simulink model "prob1"  (R2020b)
settings: Solver=VariableStepAuto  StartTime=0.0  StopTime=inf  RelTol=1e-3
settings Model: Creator=HP  LastModifiedBy=Admin

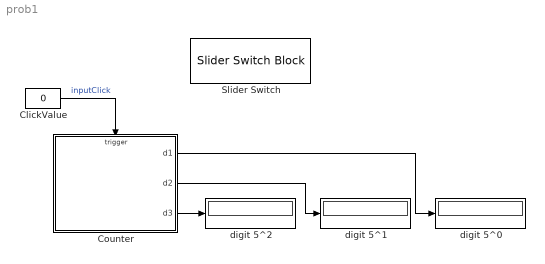
== system prob1 ==
  ClickValue : Constant  Value=0
  Counter : Stateflow chart  TreatAsAtomicUnit=on
  Slider Switch : SliderSwitchBlock  LabelPosition=Bottom
      settings: Values={{'Off', 'On'}, [0 1]}
  digit 5^0 : Display
  digit 5^1 : Display
  digit 5^2 : Display
  wires:
  Counter/1(d1) -> digit 5^0/1
  Counter/3(d3) -> digit 5^2/1
  Counter/2(d2) -> digit 5^1/1
  ClickValue/1 -> Counter/Trigger  "inputClick"

== stateflow chart prob1/Counter ==
  settings: executeAtInitialization=1
  state digit1 [parallel]
    settings: executionOrder=1
    state one
      en: d1 = 1;
    state two
      en: d1 = 2;
    state zero
      en: d1 = 0;
    state four
      en: d1 = 4;
    state three
      en: d1 = 3;
    digit1.zero -> digit1.one : inputClick
    digit1.one -> digit1.two : inputClick
    (default) -> digit1.zero
    digit1.four -> digit1.zero : inputClick /{digit2.inc2;}
    digit1.two -> digit1.three : inputClick
    digit1.three -> digit1.four : inputClick
  state digit2 [parallel]
    settings: executionOrder=2
    state one
      en: d2 = 1;
    state two
      en: d2 = 2;
    state zero
      en: d2 = 0;
    state four
      en: d2 = 4;
    state three
      en: d2 = 3;
    digit2.zero -> digit2.one : inc2
    digit2.one -> digit2.two : inc2
    (default) -> digit2.zero
    digit2.four -> digit2.zero : inc2 /{digit3.inc3;}
    digit2.two -> digit2.three : inc2
    digit2.three -> digit2.four : inc2
  state digit3 [parallel]
    settings: executionOrder=3
    state one
      en: d3 = 1;
    state two
      en: d3 = 2;
    state zero
      en: d3 = 0;
    state four
      en: d3 = 4;
    state three
      en: d3 = 3;
    digit3.zero -> digit3.one : inc3
    digit3.one -> digit3.two : inc3
    (default) -> digit3.zero
    digit3.four -> digit3.zero : inc3
    digit3.two -> digit3.three : inc3
    digit3.three -> digit3.four : inc3
  data: d1 output size=1; d2 output size=1; d3 output size=1
  events: inc2 local EITHER_EDGE_EVENT; inc3 local EITHER_EDGE_EVENT; inputClick input EITHER_EDGE_EVENT
